simulink model "BLDC_120deg_calibration_routine"  (R2024a)
settings: Solver=ode15s  StartTime=0.0  StopTime=2.25  RelTol=1e-3
model workspace (MAT data in the model file):
  t = 3
values from neighbouring files (symbols this model uses):
  D_m = 1e-3    (= 0.001)    [BLDC_Parameters.m]
  J_t = 1e-3    (= 0.001)    [BLDC_Parameters.m]
  L_ss = tau_s * r_s    (= 0.0003657)    [BLDC_Parameters.m]
  lambda_m = torque_const/(3*P/4)    (= 0.00985)    [BLDC_Parameters.m]
  P = 8    [BLDC_Parameters.m]
  r_s = r_pp/2    (= 0.345)    [BLDC_Parameters.m]
  R_vs = 1e6    (= 1000000)    [BLDC_Parameters.m]
  state1_tau = -1*mean(out.tau_state_1(end-5:end))*omega    [filter.m]
  state2_tau = -1*mean(out.tau_state_2(end-5:end))*omega    [filter.m]
  state3_tau = -1*mean(out.tau_state_3(end-5:end))*omega    [filter.m]
  state4_tau = -1*mean(out.tau_state_4(end-5:end))*omega    [filter.m]
  state5_tau = -1*mean(out.tau_state_5(end-5:end))*omega    [filter.m]
  state6_tau = -1*mean(out.tau_state_6(end-5:end))*omega    [filter.m]
  tau_s = 1.06e-3    (= 0.00106)    [BLDC_Parameters.m]
  V_bus = 12    [BLDC_Parameters.m]
undefined symbols (not defined in the file or in its folder): DiscIntNeverNeededParam, HallError1, HallError2, HallError3, WrappedHallError1
libraries: simulink x17, dspstat3 x6, spsMosfetLib x6, dspswit3 x5, spsSeriesRLCBranchLib x4, spsVoltageMeasurementLib x3, spsControlledCurrentSourceLib x3, slpidlib x1, spsPWMGeneratorDCDCLib x1, spsDCVoltageSourceLib x1, sps_lib x1
(part 2 of 2)

== system BLDC_120deg_calibration_routine/Filter1/Filter/Triggered Subsystem5 ==
  tau_curr : Inport
  tau_next : Inport  Port=2
  Trigger : TriggerPort  VariantControl=(inherit)
  Cast To Double : DataTypeConversion  OutDataTypeStr=double  SaturateOnIntegerOverflow=off  RndMeth=Floor
  Cast To Double1 : DataTypeConversion  OutDataTypeStr=double  SaturateOnIntegerOverflow=off  RndMeth=Floor
  Data Store Write : DataStoreWrite  DataStoreName=tau_curr  IndexOptions=Index vector (dialog)  Indices=1  OutputSizes=1
  Data Store Write1 : DataStoreWrite  DataStoreName=tau_next  IndexOptions=Index vector (dialog)  Indices=1  OutputSizes=1
  wires:
  tau_curr/1 -> Cast To Double/1
  Cast To Double/1 -> Data Store Write/1
  tau_next/1 -> Cast To Double1/1
  Cast To Double1/1 -> Data Store Write1/1

== system BLDC_120deg_calibration_routine/Filter/Filter/SW Trigger/Update curr_tau ==
  Data Store Read : DataStoreRead  DataStoreName=tau_next  IndexOptions=Index vector (dialog)  Indices=1  OutputSizes=1
  Data Store Write : DataStoreWrite  DataStoreName=tau_curr  IndexOptions=Index vector (dialog)  Indices=1  OutputSizes=1
  wires:
  Data Store Read/1 -> Data Store Write/1

== system BLDC_120deg_calibration_routine/Filter/Filter/SW Trigger/filtered_signals ==
  Cast To Boolean : DataTypeConversion  OutDataTypeStr=boolean  SaturateOnIntegerOverflow=off  RndMeth=Floor
  Cast To Boolean1 : DataTypeConversion  OutDataTypeStr=boolean  SaturateOnIntegerOverflow=off  RndMeth=Floor
  Cast To Boolean2 : DataTypeConversion  OutDataTypeStr=boolean  SaturateOnIntegerOverflow=off  RndMeth=Floor
  Data Store Read1 : DataStoreRead  DataStoreName=currHall  IndexOptions=Index vector (dialog)  Indices=1  OutputSizes=1
  Data Store Write1 : DataStoreWrite  DataStoreName=currHall  IndexOptions=Index vector (dialog)  Indices=1  OutputSizes=1
  MATLAB Function : MATLAB Function  TreatAsAtomicUnit=on
  Scope : Scope  NumInputPorts=5
  Scope1 : Scope  NumInputPorts=3
  Out3 : Outport
  Out2 : Outport  Port=2
  y : Outport  Port=3
  wires:
  Data Store Read1/1 -> Scope/4, MATLAB Function/1(hall_state)
  MATLAB Function/4(hall_state_next) -> Scope/5, Data Store Write1/1
  Cast To Boolean/1 -> Scope1/1, y/1
  Cast To Boolean1/1 -> Scope1/2, Out2/1
  MATLAB Function/2(H2) -> Scope/2, Cast To Boolean1/1
  MATLAB Function/3(H3) -> Scope/3, Cast To Boolean2/1
  Cast To Boolean2/1 -> Scope1/3, Out3/1
  MATLAB Function/1(H1) -> Scope/1, Cast To Boolean/1

== system BLDC_120deg_calibration_routine/Filter/Filter/SW Trigger/update next_tau ==
  Constant : Constant  Value=-1
  Data Store Write : DataStoreWrite  DataStoreName=tau_next  IndexOptions=Index vector (dialog)  Indices=1  OutputSizes=1
  wires:
  Constant/1 -> Data Store Write/1

== system BLDC_120deg_calibration_routine/Filter/Filter/Triggered Subsystem4/Subsystem ==
  In1 : Inport
  tau-1 : Inport  Port=2
  tau2 : Inport  Port=3
  tau3 : Inport  Port=4
  tau4 : Inport  Port=5
  tau-5 : Inport  Port=6
  time : Inport  Port=7
  Correction Interval : MATLAB Function  TreatAsAtomicUnit=on
  Data Store Read2 : DataStoreRead  DataStoreName=tau_curr  IndexOptions=Index vector (dialog)  Indices=1  OutputSizes=1
  Data Store Read3 : DataStoreRead  DataStoreName=tau_next  IndexOptions=Index vector (dialog)  Indices=1  OutputSizes=1
  MATLAB Function : MATLAB Function  TreatAsAtomicUnit=on
  Scope3 : Scope
  tau_corr : Outport
  Output : Outport  Port=2
  Output1 : Outport  Port=3
  wires:
  time/1 -> Correction Interval/6(time), MATLAB Function/4(time)
  Data Store Read2/1 -> MATLAB Function/2(tau_curr)
  Data Store Read3/1 -> MATLAB Function/3(tau_next)
  Correction Interval/1(tau_corr) -> Scope3/1, tau_corr/1  "tau_corr"
  MATLAB Function/1(tau_curr_out) -> Output/1
  Correction Interval/2(tau_next) -> MATLAB Function/1(tau)
  MATLAB Function/2(tau_next_out) -> Output1/1
  tau-1/1 -> Correction Interval/1(tau_1)
  tau2/1 -> Correction Interval/2(tau2)
  tau3/1 -> Correction Interval/3(tau3)
  tau4/1 -> Correction Interval/4(tau4)
  tau-5/1 -> Correction Interval/5(tau_5)

== system BLDC_120deg_calibration_routine/Filter1/Filter/Subsystem/Triggered Subsystem2 ==
  tau_curr : Inport
  tau_next : Inport  Port=2
  Trigger : TriggerPort  VariantControl=(inherit)
  Cast To Double : DataTypeConversion  OutDataTypeStr=double  SaturateOnIntegerOverflow=off  RndMeth=Floor
  Cast To Double1 : DataTypeConversion  OutDataTypeStr=double  SaturateOnIntegerOverflow=off  RndMeth=Floor
  Data Store Write : DataStoreWrite  DataStoreName=tau_curr  IndexOptions=Index vector (dialog)  Indices=1  OutputSizes=1
  Data Store Write1 : DataStoreWrite  DataStoreName=tau_next  IndexOptions=Index vector (dialog)  Indices=1  OutputSizes=1
  wires:
  tau_curr/1 -> Cast To Double/1
  Cast To Double/1 -> Data Store Write/1
  tau_next/1 -> Cast To Double1/1
  Cast To Double1/1 -> Data Store Write1/1

== system BLDC_120deg_calibration_routine/Filter1/Filter/Subsystem1/Triggered Subsystem2 ==
  tau_curr : Inport
  tau_next : Inport  Port=2
  Trigger : TriggerPort  VariantControl=(inherit)
  Cast To Double : DataTypeConversion  OutDataTypeStr=double  SaturateOnIntegerOverflow=off  RndMeth=Floor
  Cast To Double1 : DataTypeConversion  OutDataTypeStr=double  SaturateOnIntegerOverflow=off  RndMeth=Floor
  Data Store Write : DataStoreWrite  DataStoreName=tau_curr  IndexOptions=Index vector (dialog)  Indices=1  OutputSizes=1
  Data Store Write1 : DataStoreWrite  DataStoreName=tau_next  IndexOptions=Index vector (dialog)  Indices=1  OutputSizes=1
  wires:
  tau_curr/1 -> Cast To Double/1
  Cast To Double/1 -> Data Store Write/1
  tau_next/1 -> Cast To Double1/1
  Cast To Double1/1 -> Data Store Write1/1

== system BLDC_120deg_calibration_routine/Filter1/Filter/Triggered Subsystem1/Subsystem ==
  Data Store Read : DataStoreRead  DataStoreName=tau_next  IndexOptions=Index vector (dialog)  Indices=1  OutputSizes=1
  Data Store Write : DataStoreWrite  DataStoreName=tau_curr  IndexOptions=Index vector (dialog)  Indices=1  OutputSizes=1
  wires:
  Data Store Read/1 -> Data Store Write/1

== system BLDC_120deg_calibration_routine/Filter1/Filter/Triggered Subsystem1/Subsystem1 ==
  Constant : Constant  Value=-1
  Data Store Write : DataStoreWrite  DataStoreName=tau_next  IndexOptions=Index vector (dialog)  Indices=1  OutputSizes=1
  wires:
  Constant/1 -> Data Store Write/1

== system BLDC_120deg_calibration_routine/Filter1/Filter/Triggered Subsystem1/Subsystem2 ==
  Cast To Boolean : DataTypeConversion  OutDataTypeStr=boolean  SaturateOnIntegerOverflow=off  RndMeth=Floor
  Cast To Boolean1 : DataTypeConversion  OutDataTypeStr=boolean  SaturateOnIntegerOverflow=off  RndMeth=Floor
  Cast To Boolean2 : DataTypeConversion  OutDataTypeStr=boolean  SaturateOnIntegerOverflow=off  RndMeth=Floor
  Data Store Read1 : DataStoreRead  DataStoreName=currHall  IndexOptions=Index vector (dialog)  Indices=1  OutputSizes=1
  Data Store Write1 : DataStoreWrite  DataStoreName=currHall  IndexOptions=Index vector (dialog)  Indices=1  OutputSizes=1
  MATLAB Function : MATLAB Function  TreatAsAtomicUnit=on
  Scope : Scope  NumInputPorts=5
  Scope1 : Scope  NumInputPorts=3
  Out3 : Outport
  Out2 : Outport  Port=2
  y : Outport  Port=3
  wires:
  Data Store Read1/1 -> Scope/4, MATLAB Function/1(hall_state)
  MATLAB Function/4(hall_state_next) -> Scope/5, Data Store Write1/1
  Cast To Boolean/1 -> Scope1/1, y/1
  Cast To Boolean1/1 -> Scope1/2, Out2/1
  MATLAB Function/2(H2) -> Scope/2, Cast To Boolean1/1
  MATLAB Function/3(H3) -> Scope/3, Cast To Boolean2/1
  Cast To Boolean2/1 -> Scope1/3, Out3/1
  MATLAB Function/1(H1) -> Scope/1, Cast To Boolean/1

== system BLDC_120deg_calibration_routine/Filter1/Filter/Triggered Subsystem4/Subsystem ==
  In1 : Inport
  tau-1 : Inport  Port=2
  tau2 : Inport  Port=3
  tau3 : Inport  Port=4
  tau4 : Inport  Port=5
  tau-5 : Inport  Port=6
  time : Inport  Port=7
  Correction Interval : MATLAB Function  TreatAsAtomicUnit=on
  Data Store Read2 : DataStoreRead  DataStoreName=tau_curr  IndexOptions=Index vector (dialog)  Indices=1  OutputSizes=1
  Data Store Read3 : DataStoreRead  DataStoreName=tau_next  IndexOptions=Index vector (dialog)  Indices=1  OutputSizes=1
  MATLAB Function : MATLAB Function  TreatAsAtomicUnit=on
  Scope3 : Scope
  tau_corr : Outport
  Output : Outport  Port=2
  Output1 : Outport  Port=3
  wires:
  time/1 -> Correction Interval/6(time), MATLAB Function/4(time)
  Data Store Read2/1 -> MATLAB Function/2(tau_curr)
  Data Store Read3/1 -> MATLAB Function/3(tau_next)
  Correction Interval/1(tau_corr) -> Scope3/1, tau_corr/1  "tau_corr"
  MATLAB Function/1(tau_curr_out) -> Output/1
  Correction Interval/2(tau_next) -> MATLAB Function/1(tau)
  MATLAB Function/2(tau_next_out) -> Output1/1
  tau-1/1 -> Correction Interval/1(tau_1)
  tau2/1 -> Correction Interval/2(tau2)
  tau3/1 -> Correction Interval/3(tau3)
  tau4/1 -> Correction Interval/4(tau4)
  tau-5/1 -> Correction Interval/5(tau_5)

== matlab function BLDC_120deg_calibration_routine/Filter/Filter/Triggered Subsystem4/Subsystem/Correction Interval ==
  data: tau_1 input; tau2 input; tau3 input; tau_corr output; tau4 input; tau_5 input; time input; tau_next output
function [tau_corr,tau_next] = fcn(tau_1, tau2, tau3, tau4, tau_5, time)

% tau_corr = 1/3*(tau2 + 2*tau3);
tau_corr = 1/3*(4*tau_1 - tau2 + 2*tau3 - 4*tau4 + 2*tau_5);
tau_next = time + tau_corr;

== matlab function BLDC_120deg_calibration_routine/Filter/Filter/Triggered Subsystem4/Subsystem/MATLAB Function ==
  data: tau input; tau_curr_out output; tau_curr input; tau_next input; tau_next_out output; time input
function [tau_curr_out,tau_next_out] = fcn(tau, tau_curr, tau_next, time)

time = double(time);
tau_curr = double(tau_curr);

if time < tau_curr
    tau_next_out = double(tau);
    tau_curr_out = double(tau_curr);

else
    tau_curr_out = double(tau);
    tau_next_out = double(tau_next);
end

== matlab function BLDC_120deg_calibration_routine/Filter/Filter/Triggered Subsystem3/MATLAB Function ==
  data: u input; y output
function y = fcn(u)

if u == 1
    y=2;
elseif u == 2
    y=1;
elseif u == 3
    y=3;
elseif u == 4
    y=4; 
elseif u == 5
    y=6;
else
    y=5;

end

== matlab function BLDC_120deg_calibration_routine/Filter/MATLAB Function ==
  data: enable input; y output; LUT_Trigger input
function y = fcn(enable, LUT_Trigger)

y = enable & LUT_Trigger;

== matlab function BLDC_120deg_calibration_routine/Filter1/Filter/Subsystem1/Correction Interval ==
  data: tau_corr output; tau1 input; tau2 input; tau3 input; time input; tau_next output
function [tau_corr,tau_next] = fcn(tau1, tau2, tau3, time)

tau_corr = 1/3*(tau1 + tau2 + tau3);
tau_next = time + tau_corr;

== matlab function BLDC_120deg_calibration_routine/K ==
  data: Vas input; Vqs output; Vbs input; Vcs input; Vds output; theta_r input
function [Vqs, Vds] = fcn(Vas, Vbs, Vcs, theta_r)
offset = 2*pi/3;
k = (2/3)*[cos(theta_r), cos(theta_r - offset), cos(theta_r + offset);
           sin(theta_r), sin(theta_r - offset), sin(theta_r + offset)];

qds_voltage = k * [Vas; Vbs; Vcs];

Vqs = qds_voltage(1);
Vds = qds_voltage(2);

end

== matlab function BLDC_120deg_calibration_routine/Filter1/Filter/Subsystem1/MATLAB Function ==
  data: tau input; tau_curr_out output; tau_curr input; tau_next input; tau_next_out output; time input
function [tau_curr_out,tau_next_out] = fcn(tau, tau_curr, tau_next, time)

time = double(time);
tau_curr = double(tau_curr);

if time < tau_curr
    tau_next_out = double(tau);
    tau_curr_out = double(tau_curr);

else
    tau_curr_out = double(tau);
    tau_next_out = double(tau_next);
end

== matlab function BLDC_120deg_calibration_routine/Filter1/Filter/Triggered Subsystem1/Subsystem2/MATLAB Function ==
  data: hall_state input; H1 output; H2 output; H3 output; hall_state_next output
function [H1,H2,H3, hall_state_next] = fcn(hall_state)

if hall_state == 1
    H1 = 0;
    H2 = 1;
    H3 = 1;
    hall_state_next = 5;
elseif hall_state == 3
    H1 = 0;
    H2 = 1;
    H3 = 0;
    hall_state_next = 1;
elseif hall_state == 2
    H1 = 1;
    H2 = 1;
    H3 = 0;
    hall_state_next = 3;
elseif hall_state == 6
    H1 = 1;
    H2 = 0;
    H3 = 0;
    hall_state_next = 2;
elseif hall_state == 4
    H1 = 1;
    H2 = 0;
    H3 = 1;
    hall_state_next = 6;
else
    H1 = 0;
    H2 = 0;
    H3 = 1;
    hall_state_next = 4;
end

== matlab function BLDC_120deg_calibration_routine/Filter1/Filter/Triggered Subsystem4/Subsystem/Correction Interval ==
  data: tau_1 input; tau2 input; tau3 input; tau_corr output; tau4 input; tau_5 input; time input; tau_next output
function [tau_corr,tau_next] = fcn(tau_1, tau2, tau3, tau4, tau_5, time)

tau_corr = 1/3*(tau2 + 2*tau3);
tau_next = time + tau_corr;

== matlab function BLDC_120deg_calibration_routine/Filter1/Filter/Triggered Subsystem4/Subsystem/MATLAB Function ==
  data: tau input; tau_curr_out output; tau_curr input; tau_next input; tau_next_out output; time input
function [tau_curr_out,tau_next_out] = fcn(tau, tau_curr, tau_next, time)

time = double(time);
tau_curr = double(tau_curr);

if time < tau_curr
    tau_next_out = double(tau);
    tau_curr_out = double(tau_curr);

else
    tau_curr_out = double(tau);
    tau_next_out = double(tau_next);
end

== matlab function BLDC_120deg_calibration_routine/Filter/Filter/Triggered Subsystem2/MATLAB Function ==
  data: tau1 input; tau_LUT output; tau2 input; tau3 input; tau4 input; tau5 input; tau6 input; state input; time input; tau_next output
function [tau_LUT,tau_next] = fcn(tau1, tau2, tau3, tau4, tau5, tau6, state, time)

if state == 1
    tau_LUT = tau1;
elseif state == 2
    tau_LUT = tau2;
elseif state == 3
    tau_LUT = tau3;
elseif state == 4
    tau_LUT = tau4;
elseif state == 5
    tau_LUT = tau5;
else
    tau_LUT = tau6;
end

tau_next = tau_LUT + time;

== matlab function BLDC_120deg_calibration_routine/Filter/Filter/Triggered Subsystem2/MATLAB Function1 ==
  data: tau input; tau_curr_out output; tau_curr input; tau_next input; tau_next_out output; time input
function [tau_curr_out,tau_next_out] = fcn(tau, tau_curr, tau_next, time)

time = double(time);
tau_curr = double(tau_curr);

if (tau_curr > 8000)
    tau_curr = -1;
    tau_next = -1;
end

if time < tau_curr
    tau_next_out = double(tau);
    tau_curr_out = double(tau_curr);

else
    tau_curr_out = double(tau);
    tau_next_out = double(tau_next);
end

== matlab function BLDC_120deg_calibration_routine/K_inverse ==
  data: theta_r input; ias output; iqs input; ids input; ibs output; ics output
function [ias, ibs, ics] = fcn(theta_r, iqs, ids)
offset = 2*pi/3;
k_inverse = [cos(theta_r), sin(theta_r);
             cos(theta_r - offset), sin(theta_r - offset);
             cos(theta_r + offset), sin(theta_r + offset)];

abc_currents = k_inverse * [iqs; ids];

ias = abc_currents(1);
ibs = abc_currents(2);
ics = abc_currents(3);

end

== matlab function BLDC_120deg_calibration_routine/Angle Wrap ==
  data: theta_e input; wrapped_theta output
function wrapped_theta = fcn(theta_e)

wrapped_theta = wrapTo2Pi(theta_e) * 180 / pi;

== matlab function BLDC_120deg_calibration_routine/Hall Sensors3/MATLAB Function1 ==
  data: data1 input; y output; data2 input; error input
function y = fcn(data1, data2, error)

if error > 0
    y = data2;

else 
    y = data1;

end

== matlab function BLDC_120deg_calibration_routine/Filter1/Filter/Subsystem/Correction Interval ==
  data: tau_corr output; tau1 input; tau2 input; tau3 input; time input; tau_next output
function [tau_corr,tau_next] = fcn(tau1, tau2, tau3, time)

tau_corr = 1/3*(tau1 + tau2 + tau3);
tau_next = time + tau_corr;

== matlab function BLDC_120deg_calibration_routine/controller_120 ==
  data: H1 input; HALL_STATE output; H2 input; H3 input; T_vec output
function [HALL_STATE, T_vec] = controller_6step_120_sim(H1,H2,H3)
[HALL_STATE, T_vec] = controller_6step_120(H1,H2,H3);
end

== matlab function BLDC_120deg_calibration_routine/Hall Sensors3/MATLAB Function ==
  data: data1 input; y output; data2 input; error input
function y = fcn(data1, data2, error)

if error > 0
    y = data2;

else 
    y = data1;

end

== matlab function BLDC_120deg_calibration_routine/Filter/Filter/SW Trigger/filtered_signals/MATLAB Function ==
  data: hall_state input; H1 output; H2 output; H3 output; hall_state_next output
function [H1,H2,H3, hall_state_next] = fcn(hall_state)

if hall_state == 1
    H1 = 0;
    H2 = 1;
    H3 = 1;
    hall_state_next = 5;
elseif hall_state == 3
    H1 = 0;
    H2 = 1;
    H3 = 0;
    hall_state_next = 1;
elseif hall_state == 2
    H1 = 1;
    H2 = 1;
    H3 = 0;
    hall_state_next = 3;
elseif hall_state == 6
    H1 = 1;
    H2 = 0;
    H3 = 0;
    hall_state_next = 2;
elseif hall_state == 4
    H1 = 1;
    H2 = 0;
    H3 = 1;
    hall_state_next = 6;
else
    H1 = 0;
    H2 = 0;
    H3 = 1;
    hall_state_next = 4;
end

== matlab function BLDC_120deg_calibration_routine/Filter1/Filter/Subsystem/MATLAB Function ==
  data: tau input; tau_curr_out output; tau_curr input; tau_next input; tau_next_out output; time input
function [tau_curr_out,tau_next_out] = fcn(tau, tau_curr, tau_next, time)

time = double(time);
tau_curr = double(tau_curr);

if time < tau_curr
    tau_next_out = double(tau);
    tau_curr_out = double(tau_curr);

else
    tau_curr_out = double(tau);
    tau_next_out = double(tau_next);
end
